simulink model "Battery_Pack_Thermal_Management"  (R2021b)
settings: Solver=ode23t  StartTime=0.0  StopTime=2400  MaxStep=0.05  RelTol=1e-3  AbsTol=1e-3
PreLoadFcn:
  | Battery_Pack_Thermal_Management_param
undefined symbols (not defined in the file): ambient, coolantTemp, R12, R23, R34, R45, R56, R67, R78
libraries: nesl_utility x35, fl_lib x10, batteryModule_lib x8, ee_lib x1
(part 2 of 2)

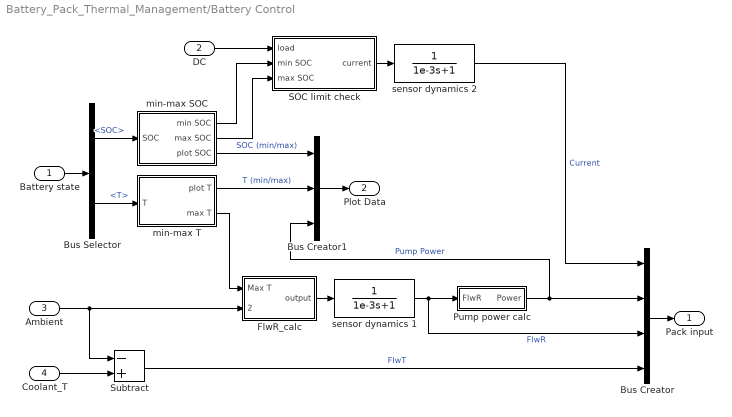
== system Battery_Pack_Thermal_Management/Battery Control ==
  Battery state : Inport
  DC : Inport  Port=2  Unit=A
  Ambient : Inport  Port=3  Unit=K
  Coolant_T : Inport  Port=4  Unit=K
  Bus Creator : BusCreator  Inputs=4
  Bus Creator1 : BusCreator  Inputs=3
  Bus Selector : BusSelector  OutputSignals=SOC,T
  FlwR_calc : Subsystem
  Pump power calc : Subsystem
  SOC limit check : Subsystem
  Subtract : Sum  Inputs=-+
  min-max SOC : Subsystem
  min-max T : Subsystem
  sensor dynamics 1 : TransferFcn  Denominator=[1e-3 1]
  sensor dynamics 2 : TransferFcn  Denominator=[1e-3 1]
  Pack input : Outport
  Plot Data : Outport  Port=2
  wires:
  SOC limit check/1(current) -> sensor dynamics 2/1
  sensor dynamics 1/1 -> Bus Creator/3, Pump power calc/1(FlwR)  "FlwR"
  min-max SOC/3(plot SOC) -> Bus Creator1/1  "SOC (min/max)"
  min-max SOC/1(min SOC) -> SOC limit check/2(min SOC)
  Bus Selector/2 -> min-max T/1(T)  "<T>"
  min-max T/1(plot T) -> Bus Creator1/2  "T (min/max)"
  sensor dynamics 2/1 -> Bus Creator/1  "Current"
  DC/1 -> SOC limit check/1(load)
  min-max SOC/2(max SOC) -> SOC limit check/3(max SOC)
  min-max T/2(max T) -> FlwR_calc/1(Max T)
  Ambient/1 -> Subtract/1, FlwR_calc/2(Ambient)
  FlwR_calc/1(output) -> sensor dynamics 1/1
  Bus Creator/1 -> Pack input/1
  Battery state/1 -> Bus Selector/1
  Bus Selector/1 -> min-max SOC/1(SOC)  "<SOC>"
  Bus Creator1/1 -> Plot Data/1
  Subtract/1 -> Bus Creator/4  "FlwT"
  Pump power calc/1(Power) -> Bus Creator1/3, Bus Creator/2  "Pump Power"
  Coolant_T/1 -> Subtract/2

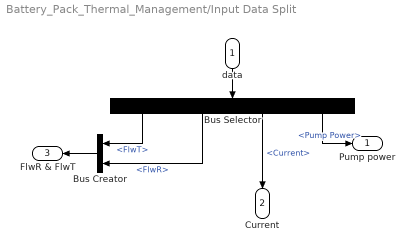
== system Battery_Pack_Thermal_Management/Input Data Split ==
  data : Inport
  Bus Creator : BusCreator  Inputs=2
  Bus Selector : BusSelector  OutputSignals=FlwT,FlwR,Current,Pump Power
  Pump power : Outport
  Current : Outport  Port=2
  FlwR & FlwT : Outport  Port=3
  wires:
  data/1 -> Bus Selector/1
  Bus Selector/1 -> Bus Creator/1  "<FlwT>"
  Bus Selector/2 -> Bus Creator/2  "<FlwR>"
  Bus Creator/1 -> FlwR & FlwT/1
  Bus Selector/3 -> Current/1  "<Current>"
  Bus Selector/4 -> Pump power/1  "<Pump Power>"

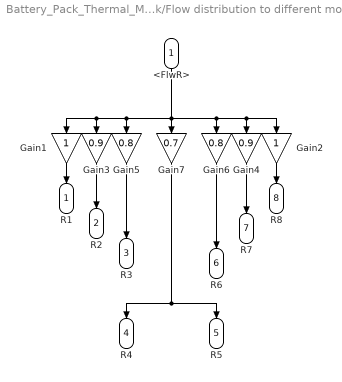
== system Battery_Pack_Thermal_Management/Battery Pack/Flow distribution to different modules ==
  <FlwR> : Inport
  Gain1 : Gain
  Gain2 : Gain
  Gain3 : Gain  Gain=0.9
  Gain4 : Gain  Gain=0.9
  Gain5 : Gain  Gain=0.8
  Gain6 : Gain  Gain=0.8
  Gain7 : Gain  Gain=0.7
  R1 : Outport
  R2 : Outport  Port=2
  R3 : Outport  Port=3
  R4 : Outport  Port=4
  R5 : Outport  Port=5
  R6 : Outport  Port=6
  R7 : Outport  Port=7
  R8 : Outport  Port=8
  wires:
  Gain4/1 -> R7/1
  Gain5/1 -> R3/1
  Gain6/1 -> R6/1
  <FlwR>/1 -> Gain1/1, Gain3/1, Gain5/1, Gain2/1, Gain4/1, Gain6/1, Gain7/1
  Gain7/1 -> R5/1, R4/1
  Gain1/1 -> R1/1
  Gain3/1 -> R2/1
  Gain2/1 -> R8/1

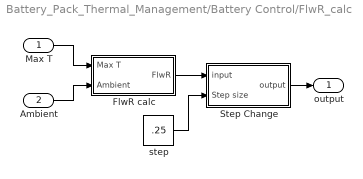
== system Battery_Pack_Thermal_Management/Battery Control/FlwR_calc ==
  Max T : Inport
  Ambient : Inport  Port=2
  FlwR calc : Subsystem
  Step Change : Subsystem
  step : Constant  Value=.25
  output : Outport
  wires:
  FlwR calc/1(FlwR) -> Step Change/1(input)
  Max T/1 -> FlwR calc/1(Max T)
  step/1 -> Step Change/2(Step size)
  Ambient/1 -> FlwR calc/2(Ambient)
  Step Change/1(output) -> output/1

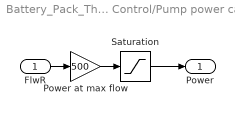
== system Battery_Pack_Thermal_Management/Battery Control/Pump power calc ==
  FlwR : Inport
  Power at max flow : Gain  Gain=500
  Saturation : Saturate  UpperLimit=500  LowerLimit=0
  Power : Outport
  wires:
  FlwR/1 -> Power at max flow/1
  Saturation/1 -> Power/1
  Power at max flow/1 -> Saturation/1

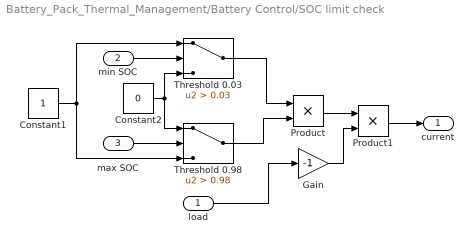
== system Battery_Pack_Thermal_Management/Battery Control/SOC limit check ==
  load : Inport
  min SOC : Inport  Port=2
  max SOC : Inport  Port=3
  Constant1 : Constant
  Constant2 : Constant  Value=0
  Gain : Gain  Gain=-1
  Product : Product
  Product1 : Product
  Threshold 0.03 : Switch  Criteria=u2 > Threshold  Threshold=0.03
  Threshold 0.98 : Switch  Criteria=u2 > Threshold  Threshold=0.98
  current : Outport
  wires:
  Constant2/1 -> Threshold 0.98/1, Threshold 0.03/3
  Product/1 -> Product1/1
  Threshold 0.98/1 -> Product/2
  load/1 -> Gain/1
  min SOC/1 -> Threshold 0.03/2
  Product1/1 -> current/1
  max SOC/1 -> Threshold 0.98/2
  Threshold 0.03/1 -> Product/1
  Gain/1 -> Product1/2
  Constant1/1 -> Threshold 0.98/3, Threshold 0.03/1

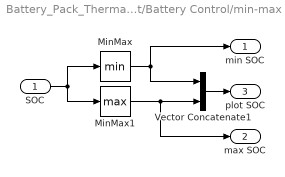
== system Battery_Pack_Thermal_Management/Battery Control/min-max SOC ==
  SOC : Inport
  MinMax : MinMax
  MinMax1 : MinMax  Function=max
  Vector Concatenate1 : Concatenate
  min SOC : Outport
  max SOC : Outport  Port=2
  plot SOC : Outport  Port=3
  wires:
  Vector Concatenate1/1 -> plot SOC/1
  SOC/1 -> MinMax1/1, MinMax/1
  MinMax/1 -> min SOC/1, Vector Concatenate1/1
  MinMax1/1 -> max SOC/1, Vector Concatenate1/2

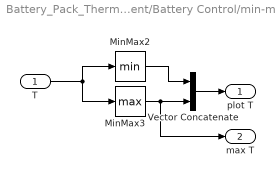
== system Battery_Pack_Thermal_Management/Battery Control/min-max T ==
  T : Inport
  MinMax2 : MinMax
  MinMax3 : MinMax  Function=max
  Vector Concatenate : Concatenate
  plot T : Outport
  max T : Outport  Port=2
  wires:
  MinMax2/1 -> Vector Concatenate/1
  Vector Concatenate/1 -> plot T/1
  MinMax3/1 -> Vector Concatenate/2, max T/1
  T/1 -> MinMax2/1, MinMax3/1

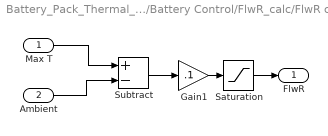
== system Battery_Pack_Thermal_Management/Battery Control/FlwR_calc/FlwR calc ==
  Max T : Inport
  Ambient : Inport  Port=2
  Gain1 : Gain  Gain=.1
  Saturation : Saturate  UpperLimit=0.95  LowerLimit=0.001
  Subtract : Sum  Inputs=+-
  FlwR : Outport
  wires:
  Subtract/1 -> Gain1/1
  Ambient/1 -> Subtract/2
  Gain1/1 -> Saturation/1
  Saturation/1 -> FlwR/1
  Max T/1 -> Subtract/1

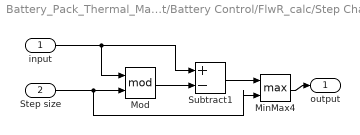
== system Battery_Pack_Thermal_Management/Battery Control/FlwR_calc/Step Change ==
  input : Inport
  Step size : Inport  Port=2
  MinMax4 : MinMax  Function=max  Inputs=2
  Mod : Math  Operator=mod  SaturateOnIntegerOverflow=on
  Subtract1 : Sum  Inputs=+-
  output : Outport
  wires:
  Mod/1 -> Subtract1/2
  MinMax4/1 -> output/1
  Subtract1/1 -> MinMax4/1
  input/1 -> Subtract1/1, Mod/1
  Step size/1 -> MinMax4/2, Mod/2
